simulink model "quad_integrator_xpc_single"  (Simulink 7.1)
settings: Solver=ode5  StartTime=0.0  StopTime=inf  FixedStep=0.0001  RelTol=1e-3
libraries: xpclib x6, xpcutilitieslib x4
settings Model: Creator=jporter  LastModifiedBy=jporter  BufferReuse=off
settings SolverCC: AutoInsertRateTranBlk=on
settings DataIOCC: LimitDataPoints=off  SaveOutput=off  SignalLogging=off  SaveTime=off
settings OptimizationCC: BlockReduction=off  OptimizeBlockIOStorage=off  BufferReuse=off  ExpressionFolding=off  LocalBlockOutputs=off
settings HardwareCC: ProdIntDivRoundTo=Zero  ProdEndianess=LittleEndian  ProdHWDeviceType=Generic->32-bit x86 compatible
settings RTWCC: SystemTargetFile=xpctarget.tlc  TemplateMakefile=xpc_default_tmf  Description=xPC Target  ProcessScript=xpctarget_make_rtw_hook
settings xpcTargetCC: TargetFcnLib=ansi_tfl_table_tmw.mat  TargetFunctionLibrary=ANSI_C  CompOptLevelCompliant=off  PortableWordSizes=off  xPCisDownloadable=off

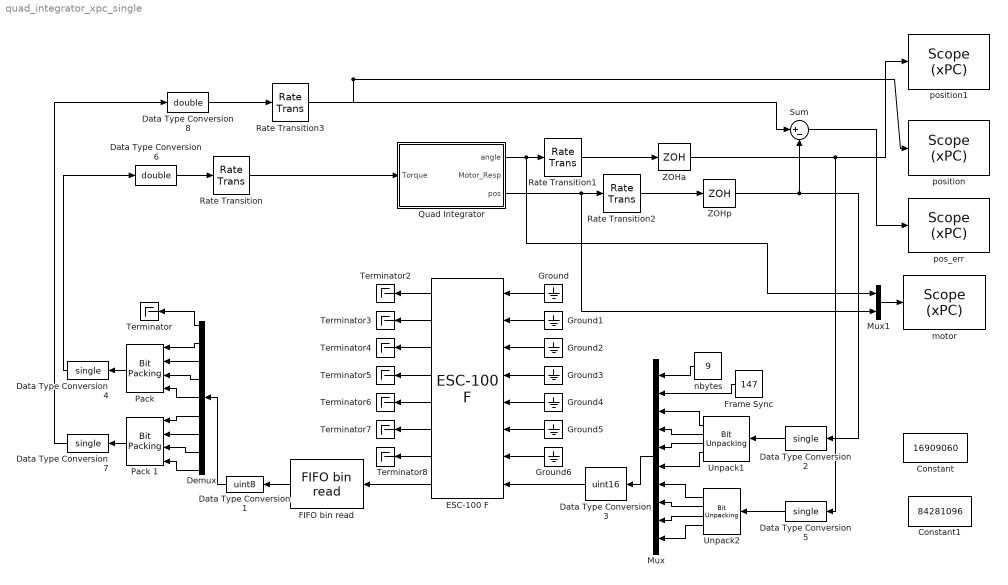
== system quad_integrator_xpc_single ==
  Constant : Constant  Orientation=left  Value=16909060  OutDataTypeMode=uint32  OutDataType=sfix(16)  OutScaling=2^0  OutDataTypeStr=uint32  SampleTime=0.02
  Constant1 : Constant  Orientation=left  Value=84281096  OutDataTypeMode=uint32  OutDataType=sfix(16)  OutScaling=2^0  OutDataTypeStr=uint32  SampleTime=0.02
  Data Type Conversion1 : DataTypeConversion  Orientation=left  OutDataTypeMode=uint8  OutDataType=sfix(16)  OutScaling=2^0  OutDataTypeStr=uint8
  Data Type Conversion{2,4..5,7} (4 alike) : DataTypeConversion  Orientation=left  OutDataTypeMode=single  OutDataType=sfix(16)  OutScaling=2^0  OutDataTypeStr=single
  Data Type Conversion3 : DataTypeConversion  Orientation=left  OutDataTypeMode=uint16  OutDataType=sfix(16)  OutScaling=2^0  OutDataTypeStr=uint16  ConvertRealWorld=Stored Integer (SI)
  Data Type Conversion6 : DataTypeConversion  OutDataTypeMode=double  OutDataType=sfix(16)  OutScaling=2^0  OutDataTypeStr=double
  Data Type Conversion8 : DataTypeConversion  OutDataTypeMode=double  OutDataType=sfix(16)  OutScaling=2^0  OutDataTypeStr=double
  Demux : Demux  Orientation=left  Outputs=9
  ESC-100 F : xpclib/RS232/Quatech/ESC-100/ESC-100 F  Orientation=left  SystemSampleTime=-1  group=FIFO Setup  port=8  irqnum=10  slot=-1  baud1=57600  parity1=None  ndata1=8  nstop1=1  fifomode1=64 deep  rlevel1=half full  automode1=off  xmtfifosize1=1024  xmtdatatype1=count+16 bit uint  rcvfifosize1=1024  baud2=57600  parity2=None  ndata2=8  nstop2=1  fifomode2=64 deep  rlevel2=half full  automode2=off  xmtfifosize2=1024  xmtdatatype2=count+16 bit uint  rcvfifosize2=1024  baud3=57600  parity3=None  ndata3=8  nstop3=1  fifomode3=64 deep  rlevel3=half full  automode3=off  xmtfifosize3=1024  xmtdatatype3=count+16 bit uint  rcvfifosize3=1024  buad4=57600  parity4=None  ndata4=8  nstop4=1  fifomode4=64 deep  rlevel4=half full  automode4=off  xmtfifosize4=1024  xmtdatatype4=count+16 bit uint  rcvfifosize4=1024  baud5=57600  parity5=None  ndata5=8  nstop5=1  fifomode5=64 deep  rlevel5=half full  automode5=off  xmtfifosize5=1024  xmtdatatype5=count+16 bit uint  rcvfifosize5=1024  baud6=57600  parity6=None  ndata6=8  nstop6=1  fifomode6=64 deep  rlevel6=half full  automode6=off  xmtfifosize6=1024  xmtdatatype6=count+16 bit uint  rcvfifosize6=1024  baud7=57600  parity7=None  ndata7=8  nstop7=1  fifomode7=64 deep  rlevel7=half full  automode7=off  xmtfifosize7=1024  xmtdatatype7=count+16 bit uint  rcvfifosize7=1024  baud8=57600  parity8=None  ndata8=8  nstop8=1  fifomode8=64 deep  rlevel8=half full  automode8=off  xmtfifosize8=1024  xmtdatatype8=count+16 bit uint  rcvfifosize8=1024
  FIFO bin read : xpclib/RS232/FIFO bin read   Orientation=left  header={char([147])}  lengths=[9]  hold=Zero output if no new data  enable=off  maxsize=9  outputtype=count+16 bit uint  sampletime=-1
  Frame Sync : Constant  Orientation=left  Value=147  OutDataTypeMode=uint8  OutDataType=sfix(16)  OutScaling=2^0  OutDataTypeStr=uint8
  Ground{,1..6} (7 alike) : Ground  Orientation=left
  Mux : Mux  Orientation=left  Inputs=10
  Mux1 : Mux  Inputs=2
  "Pack " : xpcutilitieslib/Bit Packing   Orientation=left  MaskBitPatterns={[0:7], [8:15], [16:23], [24:31]}  MaskPackDataType=single  MaskPackDataSize=[1]
  Pack 1 : xpcutilitieslib/Bit Packing   Orientation=left  MaskBitPatterns={[0:7], [8:15], [16:23], [24:31]}  MaskPackDataType=single  MaskPackDataSize=[1]
  Quad Integrator : Subsystem
  Rate Transition : RateTransition
  Rate Transition1 : RateTransition  OutPortSampleTimeOpt=Inherit  OutPortSampleTimeMultiple=2
  Rate Transition2 : RateTransition  OutPortSampleTimeOpt=Inherit  OutPortSampleTimeMultiple=2  OutPortSampleTime=0.02
  Rate Transition3 : RateTransition
  Sum : Sum  Inputs=|+-  OutDataType=sfix(16)  OutScaling=2^0
  Terminator{,2..8} (8 alike) : Terminator
  Unpack1 : xpcutilitieslib/Bit Unpacking   Orientation=left  SignExtend=off  MaskBitPatterns={[0:7], [8:15], [16:23], [24:31]}  MaskPackDataType=single  MaskPackDataSize=[1]  MaskUnpackDataTypes={'uint8', 'uint8', 'uint8', 'uint8'}  MaskUnpackDataSizes={[1], [1], [1], [1]}
  Unpack2 : xpcutilitieslib/Bit Unpacking   Orientation=left  SignExtend=off  MaskBitPatterns={[0:7], [8:15], [16:23], [24:31]}  MaskPackDataType=single  MaskPackDataSize=[1]  MaskUnpackDataTypes={'uint8', 'uint8', 'uint8', 'uint8'}  MaskUnpackDataSizes={[1], [1], [1], [1]}
  ZOHa : ZeroOrderHold  SampleTime=0.02
  ZOHp : ZeroOrderHold  SampleTime=0.02
  motor : xpclib/Misc./Scope (xPC)   SystemSampleTime=-1  scopeno=4  scopetype=Target  autostart=on  viewmode=Graphical rolling  formatstr='%15.6f'  grid=on  ylimits=[-8,8]  nosamples=200000  noprepostsamples=0  interleave=1  triggermode=FreeRun  triggersignal=1  triggerlevel=0.0  triggerslope=Either  triggerscope=1  triggersample=0  filename=data.dat  mode=Lazy  writesize=512  autorestart=off
  nbytes : Constant  Orientation=left  Value=9  OutDataTypeMode=uint8  OutDataType=sfix(16)  OutScaling=2^0  OutDataTypeStr=uint8
  pos_err : xpclib/Misc./Scope (xPC)   SystemSampleTime=-1  scopeno=3  scopetype=Target  autostart=on  viewmode=Graphical rolling  formatstr='%15.6f'  grid=on  ylimits=[-8,8]  nosamples=1000  noprepostsamples=0  interleave=1  triggermode=FreeRun  triggersignal=1  triggerlevel=0.0  triggerslope=Either  triggerscope=1  triggersample=0  filename=data.dat  mode=Lazy  writesize=512  autorestart=off
  position : xpclib/Misc./Scope (xPC)   SystemSampleTime=-1  scopeno=2  scopetype=Target  autostart=on  viewmode=Graphical rolling  formatstr='%15.6f'  grid=on  ylimits=[0,5]  nosamples=1000  noprepostsamples=0  interleave=1  triggermode=FreeRun  triggersignal=1  triggerlevel=0.0  triggerslope=Either  triggerscope=1  triggersample=0  filename=data.dat  mode=Lazy  writesize=512  autorestart=off
  position1 : xpclib/Misc./Scope (xPC)   SystemSampleTime=-1  scopeno=1  scopetype=Target  autostart=on  viewmode=Graphical rolling  formatstr='%15.6f'  grid=on  ylimits=[-1.5,1.5]  nosamples=1000  noprepostsamples=0  interleave=1  triggermode=FreeRun  triggersignal=1  triggerlevel=0.0  triggerslope=Either  triggerscope=1  triggersample=0  filename=data.dat  mode=Lazy  writesize=512  autorestart=off
  wires:
  Rate Transition/1 -> Quad Integrator/1(Torque)
  Quad Integrator/1(angle) -> Rate Transition1/1, Mux1/1
  ZOHa/1 -> Data Type Conversion5/1, position1/1
  Quad Integrator/3(pos) -> Rate Transition2/1, Mux1/2
  ZOHp/1 -> Data Type Conversion2/1, Sum/2
  Unpack1/4 -> Mux/6
  Unpack1/3 -> Mux/5
  Unpack1/2 -> Mux/4
  Unpack1/1 -> Mux/3
  Frame Sync/1 -> Mux/2
  nbytes/1 -> Mux/1
  Mux/1 -> Data Type Conversion3/1
  Demux/1 -> Terminator/1
  "Pack "/1 -> Data Type Conversion4/1
  Data Type Conversion1/1 -> Demux/1
  ESC-100 F/1 -> Terminator2/1
  ESC-100 F/2 -> Terminator3/1
  ESC-100 F/3 -> Terminator4/1
  ESC-100 F/4 -> Terminator5/1
  ESC-100 F/5 -> Terminator6/1
  ESC-100 F/6 -> Terminator7/1
  ESC-100 F/7 -> Terminator8/1
  Ground/1 -> ESC-100 F/1
  Ground1/1 -> ESC-100 F/2
  Ground2/1 -> ESC-100 F/3
  Ground3/1 -> ESC-100 F/4
  Ground4/1 -> ESC-100 F/5
  Ground5/1 -> ESC-100 F/6
  ESC-100 F/8 -> FIFO bin read/1
  Unpack2/3 -> Mux/9
  Unpack2/2 -> Mux/8
  Unpack2/1 -> Mux/7
  Unpack2/4 -> Mux/10
  FIFO bin read/1 -> Data Type Conversion1/1
  Rate Transition1/1 -> ZOHa/1
  Rate Transition2/1 -> ZOHp/1
  Data Type Conversion6/1 -> Rate Transition/1
  Data Type Conversion4/1 -> Data Type Conversion6/1
  Demux/2 -> "Pack "/1
  Demux/3 -> "Pack "/2
  Demux/4 -> "Pack "/3
  Demux/5 -> "Pack "/4
  Demux/6 -> Pack 1/1
  Demux/7 -> Pack 1/2
  Demux/8 -> Pack 1/3
  Demux/9 -> Pack 1/4
  Pack 1/1 -> Data Type Conversion7/1
  Data Type Conversion7/1 -> Data Type Conversion8/1
  Sum/1 -> pos_err/1
  Data Type Conversion8/1 -> Rate Transition3/1
  Rate Transition3/1 -> position/1, Sum/1
  Data Type Conversion2/1 -> Unpack1/1
  Data Type Conversion5/1 -> Unpack2/1
  Mux1/1 -> motor/1
  Ground6/1 -> ESC-100 F/7
  Data Type Conversion3/1 -> ESC-100 F/8

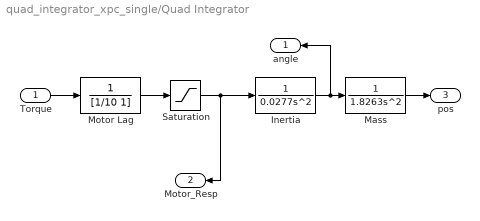
== system quad_integrator_xpc_single/Quad Integrator ==
  Torque : Inport
  Inertia : TransferFcn  Denominator=[0.0277 0 0]
  Mass : TransferFcn  Denominator=[1.8263 0 0]
  Motor Lag : TransferFcn  Denominator=[1/10 1]
  Saturation : Saturate  UpperLimit=40  LowerLimit=-40  OutDataType=sfix(16)  OutScaling=2^0
  angle : Outport  Orientation=left
  Motor_Resp : Outport  Orientation=left  Port=2
  pos : Outport  Port=3
  wires:
  Motor Lag/1 -> Saturation/1
  Saturation/1 -> Inertia/1, Motor_Resp/1
  Inertia/1 -> Mass/1, angle/1
  Mass/1 -> pos/1
  Torque/1 -> Motor Lag/1
